simulink subsystem "INDI"  (R2019b)
settings: Solver=VariableStepAuto  StartTime=0.0  StopTime=10.0  RelTol=1e-3
settings Model: Creator=mauro  LastModifiedBy=mauro

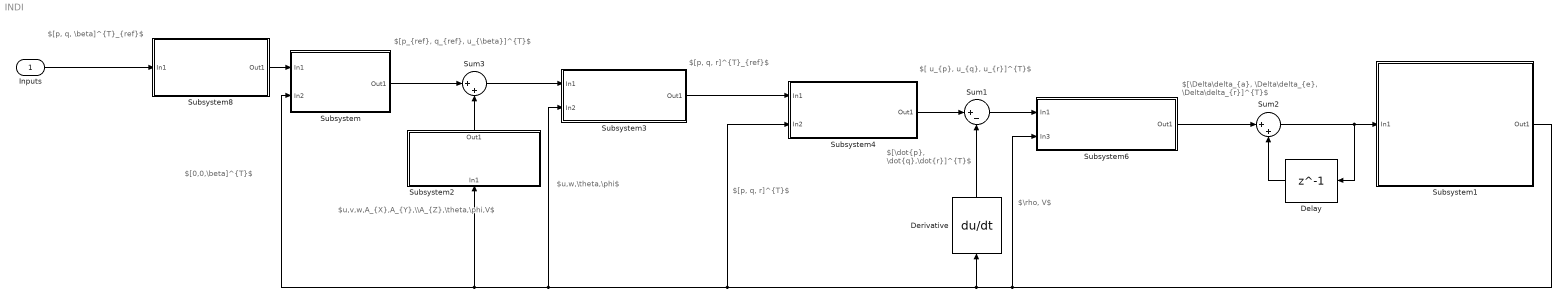
== system INDI ==
  note: $[p, q, r]^{T}_{ref}$
  note: $[p_{ref}, q_{ref}, \nu_{\beta}]^{T}$
  note: $[\nu_{p}, \nu_{q}, \nu_{r}]^{T}$
  note: $[\Delta\delta_{a}, \Delta\delta_{e}, \Delta\delta_{r}]^{T}$
  note: $\rho, V$
  note: $[0,0,\beta]^{T}$
  note: $[p, q, r]^{T}$
  note: $u,v,w,A_{X},A_{Y},\\A_{Z},\theta,\phi,V$
  note: $u,w,\theta,\phi$
  note: $[p, q, \beta]^{T}_{ref}$
  note: $[\dot{p}, \dot{q},\dot{r}]^{T}$
  Inputs : Inport
  Delay : Delay  DelayLength=1  InitialCondition=0
      mask Display: image("C:\Users\mauro\OneDrive\AE Master - TU Delft\Nonlinear and Adaptive Flight Control (AE4311)\AE4311_FTFCAssignment\cessna_model\controller_fig\z-1.png")
  Derivative : Derivative
      mask Display: image("C:\Users\mauro\OneDrive\AE Master - TU Delft\Nonlinear and Adaptive Flight Control (AE4311)\AE4311_FTFCAssignment\cessna_model\controller_fig\derv.png")
  Subsystem : Subsystem
      mask Display: image("C:\Users\mauro\OneDrive\AE Master - TU Delft\Nonlinear and Adaptive Flight Control (AE4311)\AE4311_FTFCAssignment\cessna_model\controller_fig\lc_2.png")
  Subsystem1 : Subsystem
      mask Display: image("C:\Users\mauro\OneDrive\AE Master - TU Delft\Nonlinear and Adaptive Flight Control (AE4311)\AE4311_FTFCAssignment\cessna_model\controller_fig\ac.jpg")
  Subsystem2 : Subsystem
      mask Display: image("C:\Users\mauro\OneDrive\AE Master - TU Delft\Nonlinear and Adaptive Flight Control (AE4311)\AE4311_FTFCAssignment\cessna_model\controller_fig\a_kyn.png")
  Subsystem3 : Subsystem
      mask Display: image("C:\Users\mauro\OneDrive\AE Master - TU Delft\Nonlinear and Adaptive Flight Control (AE4311)\AE4311_FTFCAssignment\cessna_model\controller_fig\b_kyn.png")
  Subsystem4 : Subsystem
      mask Display: image("C:\Users\mauro\OneDrive\AE Master - TU Delft\Nonlinear and Adaptive Flight Control (AE4311)\AE4311_FTFCAssignment\cessna_model\controller_fig\lc_1.png")
  Subsystem6 : Subsystem
      mask Display: image("C:\Users\mauro\OneDrive\AE Master - TU Delft\Nonlinear and Adaptive Flight Control (AE4311)\AE4311_FTFCAssignment\cessna_model\controller_fig\b_dyn.png")
  Subsystem8 : Subsystem
      mask Display: image("C:\Users\mauro\OneDrive\AE Master - TU Delft\Nonlinear and Adaptive Flight Control (AE4311)\AE4311_FTFCAssignment\cessna_model\controller_fig\lpf.png")
  Sum1 : Sum  Inputs=|+-
  Sum2 : Sum  Inputs=|++
  Sum3 : Sum  Inputs=|++
  wires:
  Inputs/1 -> Subsystem8/1(In1)
  Subsystem1/1(Out1) -> Subsystem/2(In2), Subsystem2/1(In1), Subsystem3/2(In2), Subsystem4/2(In2), Derivative/1, Subsystem6/2(In3)
  Subsystem/1(Out1) -> Sum3/1
  Subsystem2/1(Out1) -> Sum3/2
  Sum3/1 -> Subsystem3/1(In1)
  Subsystem3/1(Out1) -> Subsystem4/1(In1)
  Subsystem4/1(Out1) -> Sum1/1
  Derivative/1 -> Sum1/2
  Sum1/1 -> Subsystem6/1(In1)
  Subsystem6/1(Out1) -> Sum2/1
  Subsystem8/1(Out1) -> Subsystem/1(In1)
  Sum2/1 -> Subsystem1/1(In1), Delay/1
  Delay/1 -> Sum2/2

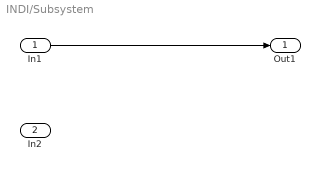
== system INDI/Subsystem ==
  In1 : Inport
  In2 : Inport  Port=2
  Out1 : Outport
  wires:
  In1/1 -> Out1/1

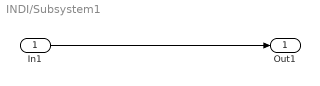
== system INDI/Subsystem1 ==
  In1 : Inport
  Out1 : Outport
  wires:
  In1/1 -> Out1/1

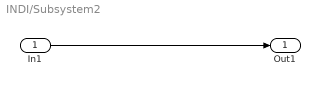
== system INDI/Subsystem2 ==
  In1 : Inport
  Out1 : Outport
  wires:
  In1/1 -> Out1/1

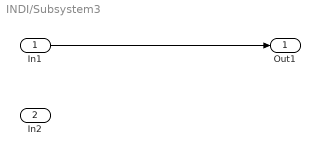
== system INDI/Subsystem3 ==
  In1 : Inport
  In2 : Inport  Port=2
  Out1 : Outport
  wires:
  In1/1 -> Out1/1

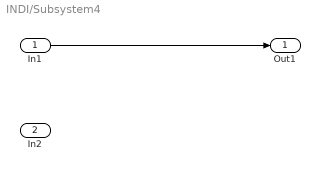
== system INDI/Subsystem4 ==
  In1 : Inport
  In2 : Inport  Port=2
  Out1 : Outport
  wires:
  In1/1 -> Out1/1

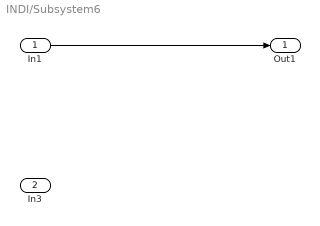
== system INDI/Subsystem6 ==
  In1 : Inport
  In3 : Inport  Port=2
  Out1 : Outport
  wires:
  In1/1 -> Out1/1

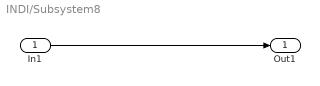
== system INDI/Subsystem8 ==
  In1 : Inport
  Out1 : Outport
  wires:
  In1/1 -> Out1/1
